simulink model "v2022_Modello_SITL_AENEA_2020b"  (R2020b)
settings: Solver=ode4  StartTime=0.0  StopTime=300  FixedStep=0.01  RelTol=1e-3
values from neighbouring files (symbols this model uses):
  alphavec_rad = [-0.10471975512 -0.0872664625997 -0.0698131700798 -0.0523598775598 -0.0349065850399 -0.0174532925199 0 0.0174532925199 0.0349065850399 0.0523598775598 0.0698131700798 0.0872664625997 ... (13 elements, 1x13)]    [datiAerodinamiciAENEA.mat]    (also in v2021_10_27_calcoloAerodinamica.m = deg2rad(alphavec))
  attuatore_Amax = 20*(pi/180)    (= 0.349065850399)    [v2021_10_27_avvioSITL.m]    (also in v2021_10_27_calcoloAerodinamica.m)
  attuatore_Emax = 25*(pi/180)    (= 0.436332312999)    [v2021_10_27_avvioSITL.m]    (also in v2021_10_27_calcoloAerodinamica.m)
  attuatore_Rmax = 25*(pi/180)    (= 0.436332312999)    [v2021_10_27_avvioSITL.m]    (also in v2021_10_27_calcoloAerodinamica.m)
  b = 2.62    [datiAerodinamiciAENEA.mat]    (also in derivateROSKAM_new.m; v2021_10_27_calcoloAerodinamica.m)
  beta_phi = 1/10.5600    (= 0.094696969697)    [Load_modello_sensori.m]
  beta_psi = 1/170    (= 0.00588235294118)    [Load_modello_sensori.m]
  beta_theta = 1/10.5000    (= 0.0952380952381)    [Load_modello_sensori.m]
  betavec_rad = [-0.209439510239 -0.13962634016 -0.0698131700798 0 0.0698131700798 0.13962634016 0.209439510239]    [datiAerodinamiciAENEA.mat]    (also in v2021_10_27_calcoloAerodinamica.m = deg2rad(betavec))
  c = 0.32    [datiAerodinamiciAENEA.mat]    (also in derivateROSKAM_new.m; v2021_10_27_calcoloAerodinamica.m)
  cbar = 0.32    [datiAerodinamiciAENEA.mat]    (also in v2021_10_27_calcoloAerodinamica.m)
  CD0 = 0.2    [datiAerodinamiciAENEA.mat]    (also in v2021_10_27_calcoloAerodinamica.m = 0.024)
  CldA = KCldA(1)*180/pi    [Alettoni.m]    (also in datiAerodinamiciAENEA.mat = 0.490103315517)
  CLdE = KCLdE(1)*180/pi    [Equilibratore.m]    (also in datiAerodinamiciAENEA.mat = 0.809101149087)
  CldR = 0.0568697125654    [datiAerodinamiciAENEA.mat]
  Clp = -0.4318    [datiAerodinamiciAENEA.mat]    (also in derivateROSKAM_new.m = clp_w+2*(Zv/b)^2*cy_betav+Clp_tail; v2021_10_27_calcoloAerodinamica.m)
  CLq = 8.13    [datiAerodinamiciAENEA.mat]    (also in v2021_10_27_calcoloAerodinamica.m)
  Clr = 0.1459    [datiAerodinamiciAENEA.mat]    (also in derivateROSKAM_new.m = cl*clr_cl-(2/b^2)*(lv*cos(alpha)+Zv*sin(alpha))*(Zv*cos(alph; v2021_10_27_calcoloAerodinamica.m)
  CmdE = KCmdE(1)*180/pi    [Equilibratore.m]    (also in datiAerodinamiciAENEA.mat = -3.59730623976)
  Cmq = -23.24    [datiAerodinamiciAENEA.mat]    (also in derivateROSKAM_new.m = -K*cL_alphaw*((AR*(2*(Xw/c)^2+0.5*(Xw/c))/(AR+2))+1/8)-2*cL_; v2021_10_27_calcoloAerodinamica.m)
  CndA = KCndA(1)*180/pi    [Alettoni.m]    (also in datiAerodinamiciAENEA.mat = -0.0456969018066)
  CndR = -0.162544523826    [datiAerodinamiciAENEA.mat]
  Cnp = 0.000294    [datiAerodinamiciAENEA.mat]    (also in derivateROSKAM_new.m = -clp_w*tan(alpha)+Clp*tan(alpha)-(2/b)*(lv*cos(alpha)+Zv*sin; v2021_10_27_calcoloAerodinamica.m = 0.007507)
  Cnr = -0.4872    [datiAerodinamiciAENEA.mat]    (also in derivateROSKAM_new.m = (Cnr_Clquadro)*cl^2+(cnr_cd0)*cd0+(2/b^2)*(lv*cos(alpha)+Zv*; v2021_10_27_calcoloAerodinamica.m)
  CYdA = KCYdA(1)*180/pi    [Alettoni.m]    (also in datiAerodinamiciAENEA.mat = -0.0146577407549)
  CYdR = -0.298131751664    [datiAerodinamiciAENEA.mat]
  CYp = 0.050728    [datiAerodinamiciAENEA.mat]    (also in v2021_10_27_calcoloAerodinamica.m)
  CYr = 0.358925    [datiAerodinamiciAENEA.mat]    (also in v2021_10_27_calcoloAerodinamica.m)
  delay_ahrs = 0    [Load_modello_sensori.m]
  delay_bmp = 0    [Load_modello_sensori.m]
  delay_gps = 0    [Load_modello_sensori.m]
  deltaAtrim = 0    [v2021_10_27_avvioSITL.m]
  deltaEtrim = (Cm0*CL_alpharad+Cm_alpharad*CLtrim)/(CL_alpharad*CmdE)    [calcoloDatiIniziali.m]    (also in v2021_10_27_avvioSITL.m = 0)
  deltaRtrim = 0    [v2021_10_27_avvioSITL.m]
  deltaTtrim = 0.1    [v2021_10_27_avvioSITL.m]
  Dprop = 0.5334    [datiAerodinamiciAENEA.mat]    (also in v2021_10_27_calcoloAerodinamica.m)
  g = [0 0 9.81]    [datiAerodinamiciAENEA.mat]    (also in v2021_10_27_calcoloAerodinamica.m = [0 0 9.81]')
  HINI = -State0.Pos0(3)    [v2021_10_27_avvioSITL.m]
  Ingaggio_AP = input("inserire 1 se si vuole ingaggiare l' AP, 0 altrimenti: ")    [v2021_10_27_avvioSITL.m]
  J_vec = [0 0.03 0.06 0.09 0.11 0.14 0.17 0.2 0.23 0.26 0.28 0.31 ... (30 elements, 30x1)]    [datiAerodinamiciAENEA.mat]
  Jeng = 0    [datiAerodinamiciAENEA.mat]    (also in v2021_10_27_calcoloAerodinamica.m)
  Jprop = 0.00422031414    [datiAerodinamiciAENEA.mat]    (also in v2021_10_27_calcoloAerodinamica.m)
  latitudineINI = 41.88754294247101*pi/180    (= 0.731075539917)    [v2021_10_27_avvioSITL.m]
  longitudineINI = 12.539364533818434*pi/180    (= 0.218853197223)    [v2021_10_27_avvioSITL.m]
  mean_ax = 0*0.0392    (= 0)    [Load_modello_sensori.m]
  mean_ay = -0*0.0598    (= 0)    [Load_modello_sensori.m]
  mean_az = 0*0.0384    (= 0)    [Load_modello_sensori.m]
  mean_p = 0*1.5184e-06    (= 0)    [Load_modello_sensori.m]
  mean_q = 0*2.9671e-05    (= 0)    [Load_modello_sensori.m]
  mean_r = 0*5.4105e-05    (= 0)    [Load_modello_sensori.m]
  P_ref = 1.0074e+05    (= 100740)    [Load_modello_sensori.m]
  PWM_Aileron = rad2deg(deltaAtrim)*9+1503    [v2021_10_27_avvioSITL.m]
  PWM_Elevator = rad2deg(deltaEtrim)*(447/50)+(3007/2)    [v2021_10_27_avvioSITL.m]
  PWM_Rudder = rad2deg(deltaRtrim)*(447/50)+(3007/2)    [v2021_10_27_avvioSITL.m]
  PWM_Throttle = (deltaTtrim)*800+1100    (= 1180)    [v2021_10_27_avvioSITL.m]
  q = prediction(11)    [f_pred_F1B.m]
  r = prediction(12)    [f_pred_F1B.m]
  rACtG = [-1.334 0 -0.2103]    [datiAerodinamiciAENEA.mat]    (also in v2021_10_27_calcoloAerodinamica.m = rACtP-rGP)
  rACwG = [-0.0589 0 -0.1645]    [datiAerodinamiciAENEA.mat]    (also in v2021_10_27_calcoloAerodinamica.m = rACwP-rGP)
  rAHRSG = [0 0 0.1075]    [datiAerodinamiciAENEA.mat]    (also in v2021_10_27_calcoloAerodinamica.m = rAHRSP-rGP)
  rho = 1.2133    [datiAerodinamiciAENEA.mat]    (also in derivateROSKAM_new.m = 1.16123787958; v2021_10_27_calcoloAerodinamica.m)
  rLEG = [0.0211 0 -0.1645]    [datiAerodinamiciAENEA.mat]    (also in v2021_10_27_calcoloAerodinamica.m = rLEP-rGP)
  rmglG = [-0.2319 -0.2 0.3925]    [datiAerodinamiciAENEA.mat]    (also in v2021_10_27_calcoloAerodinamica.m = rmglP-rGP)
  rmgrG = [-0.2319 0.2 0.3925]    [datiAerodinamiciAENEA.mat]    (also in v2021_10_27_calcoloAerodinamica.m = rmgrP-rGP)
  rngG = [0.2969 0 0.3925]    [datiAerodinamiciAENEA.mat]    (also in v2021_10_27_calcoloAerodinamica.m = rngP-rGP)
  rNPG = [-0.2442 0 -0.1645]    [datiAerodinamiciAENEA.mat]    (also in v2021_10_27_calcoloAerodinamica.m = rNPP-rGP)
  rPG = [0.5 0 -0.1075]    [datiAerodinamiciAENEA.mat]    (also in v2021_10_27_calcoloAerodinamica.m = -rGP)
  Rprop = 0.2667    [datiAerodinamiciAENEA.mat]    (also in v2021_10_27_calcoloAerodinamica.m)
  S = 0.8384    [datiAerodinamiciAENEA.mat]    (also in derivateROSKAM_new.m; v2021_10_27_calcoloAerodinamica.m)
  seed_ahrs = randi([0 2000],1,1)    [Load_modello_sensori.m]
  seed_baro = randi([0 2000],1,1)    [Load_modello_sensori.m]
  seed_gps = randi([0 2000],1,1)    [Load_modello_sensori.m]
  sensori_FreqCampionamento_pitot = 0.02    [v2021_10_27_avvioSITL.m]
  sensori_RumoreSampleTime = 0.02    [v2021_10_27_avvioSITL.m]
  sensori_varianza = 0.0000    (= 0)    [v2021_10_27_avvioSITL.m]
  Std_con_lat = 2.7349e-07    [Load_modello_sensori.m]
  Std_con_long = 1.3733e-06    [Load_modello_sensori.m]
  Std_vel = 0.05    [Load_modello_sensori.m]
  T0_ref = 25    [Load_modello_sensori.m]
  Ta_lat = 10^2    (= 100)    [Load_modello_sensori.m]
  Ta_long = 10^2    (= 100)    [Load_modello_sensori.m]
  Ts_ahrs = 0.02    [Load_modello_sensori.m]
  Ts_bmp = 0.02    [Load_modello_sensori.m]
  Ts_gps = 0.2    [Load_modello_sensori.m]
  tsamp = 0.02    [v2021_10_27_avvioSITL.m]
  V_cruise = input('inserire un valore desiderato per V_cruise: ')    [trimCalc.m]
  Var_heading_static = 0.1    [Load_modello_sensori.m]
  Var_V_hor = 0.5*0.01    (= 0.005)    [Load_modello_sensori.m]
  Var_V_hor_static = 0.25    [Load_modello_sensori.m]
  W = [0 0 92.214]    [datiAerodinamiciAENEA.mat]    (also in derivateROSKAM_new.m = 112.815; v2021_10_27_calcoloAerodinamica.m = m*g)
  White_ax = 1.486e-04    (= 0.0001486)    [Load_modello_sensori.m]
  White_ay = 9.403e-05    [Load_modello_sensori.m]
  White_az = 1.648e-04    (= 0.0001648)    [Load_modello_sensori.m]
  White_gm_phi = 3.2740e-05    (= 3.274e-05)    [Load_modello_sensori.m]
  White_gm_psi = 2.9162e-04    (= 0.00029162)    [Load_modello_sensori.m]
  White_gm_theta = 2.4704e-05    [Load_modello_sensori.m]
  White_p = 2.934e-05    [Load_modello_sensori.m]
  White_pressione = 10.18    [Load_modello_sensori.m]
  White_r = 3.258e-05    [Load_modello_sensori.m]
  WP_AL = [     0 20 0 0 41.807822 12.589274 3 ... (first row only)    [v2021_10_27_avvioSITL.m]
  WP_db_info = [0 0 0 0 1 3;              0 0 0 0 2 3;              0 0 0 0 3 3;              0 0 0 0 0 0]    [v2021_10_27_avvioSITL.m]
  WP_db_param = [              0 0 17 0 41.887798530888304, 12.537905412104232 75;              0 0 20 0 41.89052329007801, 12.492437426923948 65;              0 0 24 0 41.93506891472633, 12.504514543566634 80;              0 0 0 0 0 0 0 ... (first row only)    [v2021_10_27_avvioSITL.m]
  Zeng = -0.1075    [datiAerodinamiciAENEA.mat]    (also in v2021_10_27_calcoloAerodinamica.m = rPG(3))
  Zpista = 0    [v2021_10_27_avvioSITL.m]
undefined symbols (not defined in the file or in its folder): Earth, F, h_home, matricepolinomi, MIL, Receive, Send, State0, Var_heading, WGS84
libraries: simulink_extras x27, aerolibfltsims x5, simulink x3, aerolibwind2 x3, aerolibasang x2, shared6dof x1, slpidlib x1, aerolibatmos2 x1, aerolibanimutils x1
(part 1 of 4)
settings Model: PacingRate=0.010000  Creator=Giorgio  LastModifiedBy=User
settings DataIOCC: ReturnWorkspaceOutputs=off
settings DebuggingCC: ParameterPrecisionLossMsg=none  BusObjectLabelMismatch=none  ArithmeticOperatorsInVariantConditions=warning
settings SFSimCC: CustomCodeUndefinedFunction=UseInterfaceOnly

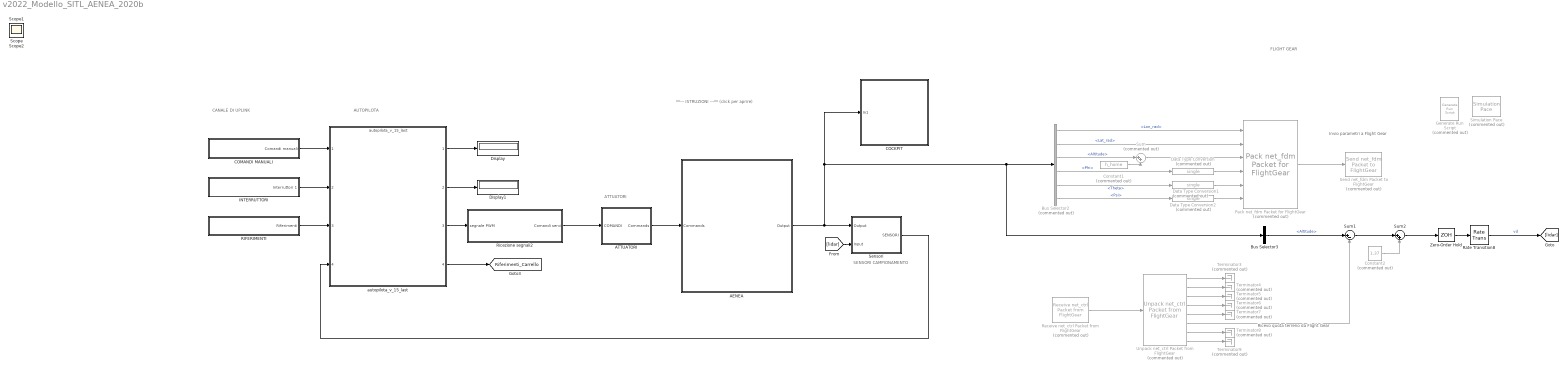
== system v2022_Modello_SITL_AENEA_2020b ==
  note: AUTOPILOTA
  note: SENSORI
      | CAMPIONAMENTO
  note: ATTUATORI
  note: CANALE DI UPLINK
  note: Ricevo quota terreno da Flight Gear
  note: Invio parametri a Flight Gear
  note: FLIGHT GEAR
  note: **--- ISTRUZIONI ---**
      | (click per aprire)
  "AENEA " : Subsystem
  ATTUATORI : Subsystem
  Bus Selector2 : BusSelector  Commented=on  OutputSignals=Lon_rad,Lat_rad,Altitude,Phi,Theta,Psi
  Bus Selector3 : BusSelector  OutputSignals=Altitude
  COCKPIT : Subsystem
  COMANDI MANUALI : Subsystem
  Constant1 : Constant  Commented=on  Value=h_home
  Constant2 : Constant  Commented=on  Value=1.37
  Data Type Conversion : DataTypeConversion  Commented=on  OutDataTypeStr=single
  Data Type Conversion1 : DataTypeConversion  Commented=on  OutDataTypeStr=single
  Data Type Conversion2 : DataTypeConversion  Commented=on  OutDataTypeStr=single
  Display : Display
  Display1 : Display
  Generate Run Script : aerolibfltsims/Generate Run Script  Commented=on  Architecture=Default  dataFlow=Send-Receive  GeometryModelName=c172p  AirportId=LIRF  RunwayId=34L  InitialAltitude=0  InitialHeading=340  OffsetDistance=0  OffsetAzimuth=0  InstallScenery=off  DisableShaders=off  OriginAddress=127.0.0.1  DestinationPort=5502  OriginPort=5505  LocalAddress=127.0.0.1  OutputFileName=runfg_sr.bat  FlightGearBaseDirectory=C:\Program Files\FlightGear 2016.1.2
  "INTERRUTTORI " : Subsystem
  Pack net_fdm Packet for FlightGear : aerolibfltsims/Pack net_fdm Packet for FlightGear  Commented=on  FlightGearVersion=v2016.1  ShowPositionAttitudeInputs=on  ShowVelocityAccelerationInputs=off  ShowControlSurfacePositionInputs=off  ShowEngineFuelInputs=off  ShowLandingGearInputs=off  ShowEnvironmentInputs=off  SampleTime=-1  packetVersion=24
      settings: SourceProductBaseCode=AE
  RIFERIMENTI : Subsystem
  Rate Transition8 : RateTransition  Deterministic=off  InitialCondition=State0.Pos0(3)  OutPortSampleTime=0.02
  Receive net_ctrl Packet from FlightGear : aerolibfltsims/Receive net_ctrl Packet from FlightGear  Commented=on  FlightGearVersion=v2016.1  ReceiveAddress=127.0.0.1  ReceivePort=5505  ReceiveWidth=744  varLen=off  SampleTime=-1  packetFlag=off
      settings: AttributesFormatString=Version Selected:\n%<FlightGearVersion>  SourceProductBaseCode=AE
  Ricezione segnali2 : Subsystem
  Send net_fdm Packet to FlightGear : aerolibfltsims/Send net_fdm Packet to FlightGear  Commented=on  DestinationIpAddress=127.0.0.1  DestinationPort=5502  LocalIpPort=-1  varLen=off  SampleTime=-1
      settings: SourceProductBaseCode=AE
  Sensori : Subsystem
  Simulation Pace : aerolibanimutils/Simulation Pace  Commented=on  SimulationPace=1  SleepMode=MATLAB Thread  OutputPaceError=off  SampleTime=tsamp
  Sum : Sum  Commented=on  Inputs=|++
  Sum1 : Sum  Inputs=|+-
  Sum2 : Sum  Inputs=|++
  Terminator{3..9} (7 alike) : Terminator  Commented=on
  Unpack net_ctrl Packet from FlightGear : aerolibfltsims/Unpack net_ctrl Packet from FlightGear  Commented=on  FlightGearVersion=v2016.1  ShowControlSurfacePositionOutputs=off  ShowEngineFuelOutputs=off  ShowLandingGearOutputs=off  ShowAvionicOutputs=off  ShowEnvironmentOutputs=on  SampleTime=-1  packetVersion=27
      settings: AttributesFormatString=Version Selected: %<FlightGearVersion>  SourceProductBaseCode=AE
  Zero-Order Hold : ZeroOrderHold  SampleTime=0.02
  autopilota_v_15_last : ModelReference  ModelNameDialog=autopilota_v_15_last.slx  SimulationMode=Normal  ModelReferenceVersion=4.21
  Scope : Scope
  Scope1 : Scope
  Scope2 : Scope
  tag scope: Riferimenti_Carrello=global
  wires:
  autopilota_v_15_last/1 -> Display/1
  "INTERRUTTORI "/1(Interruttori 1) -> autopilota_v_15_last/2
  COMANDI MANUALI/1(Comandi manuali) -> autopilota_v_15_last/1
  autopilota_v_15_last/2 -> Display1/1
  RIFERIMENTI/1(Riferimenti) -> autopilota_v_15_last/3
  Constant2/1 -> Sum2/2
  Bus Selector2/6 -> Data Type Conversion2/1  "<Psi>"
  Bus Selector2/3 -> Sum/1  "<Altitude>"
  Sum1/1 -> Sum2/1
  Unpack net_ctrl Packet from FlightGear/6 -> Sum1/2
  Unpack net_ctrl Packet from FlightGear/2 -> Terminator4/1
  Unpack net_ctrl Packet from FlightGear/7 -> Terminator8/1
  Rate Transition8/1 -> [lidar]  "vd"
  Receive net_ctrl Packet from FlightGear/1 -> Unpack net_ctrl Packet from FlightGear/1
  Sum2/1 -> Zero-Order Hold/1
  Unpack net_ctrl Packet from FlightGear/8 -> Terminator9/1
  Bus Selector2/2 -> Pack net_fdm Packet for FlightGear/2  "<Lat_rad>"
  Constant1/1 -> Sum/2
  Data Type Conversion2/1 -> Pack net_fdm Packet for FlightGear/6
  Bus Selector3/1 -> Sum1/1  "<Altitude>"
  Unpack net_ctrl Packet from FlightGear/3 -> Terminator5/1
  Pack net_fdm Packet for FlightGear/1 -> Send net_fdm Packet to FlightGear/1
  Zero-Order Hold/1 -> Rate Transition8/1
  Data Type Conversion/1 -> Pack net_fdm Packet for FlightGear/4
  Sum/1 -> Pack net_fdm Packet for FlightGear/3
  Bus Selector2/4 -> Data Type Conversion/1  "<Phi>"
  Bus Selector2/5 -> Data Type Conversion1/1  "<Theta>"
  Unpack net_ctrl Packet from FlightGear/1 -> Terminator3/1
  Data Type Conversion1/1 -> Pack net_fdm Packet for FlightGear/5
  Bus Selector2/1 -> Pack net_fdm Packet for FlightGear/1  "<Lon_rad>"
  Unpack net_ctrl Packet from FlightGear/4 -> Terminator6/1
  Unpack net_ctrl Packet from FlightGear/5 -> Terminator7/1
  [lidar] -> Sensori/2(Input)
  "AENEA "/1(Output) -> Sensori/1(Output), COCKPIT/1(In1), Bus Selector3/1, Bus Selector2/1
  ATTUATORI/1(Commands) -> "AENEA "/1(Commands)
  autopilota_v_15_last/3 -> Ricezione segnali2/1(segnale PWM)
  Ricezione segnali2/1(Comandi servi) -> ATTUATORI/1("COMANDI ")
  Sensori/1(SENSORI) -> autopilota_v_15_last/4
  autopilota_v_15_last/4 -> [Riferimenti_Carrello]

== system v2022_Modello_SITL_AENEA_2020b/AENEA  ==
  Commands : Inport  OutDataTypeStr=double
  AENEA II_SITL1 : Subsystem
  Blocco_Costanti1 : Subsystem
  Bus Creator : BusCreator  Inputs=4
  Bus Creator1 : BusCreator  Inputs=4
  Bus Selector : BusSelector  OutputSignals=deltaE,deltaA,deltaR,Manetta
  Bus Selector1 : BusSelector  OutputSignals=xyz.h
  Bus Selector2 : BusSelector  OutputSignals=Vbpolare.V
  Constant : Constant  Value=[0,0,0]
  Constant1 : Constant  Value=rho
  Constant2 : Constant  Value=1/2
  Gain : Gain  Gain=-1
  ISA Atmosphere Model : aerolibatmos2/ISA Atmosphere Model  custom=off  g=9.80665  gamma=1.4  R=287.0531  L=0.0065  h_trop=11000  h_strat=20000  rho0=1.225  P0=101325  T0=288.15  h0=0
  Product : Product  Inputs=3
  Square : Math  Operator=square  SaturateOnIntegerOverflow=on
  Terminator : Terminator
  Terminator1 : Terminator
  Terminator2 : Terminator
  toSensors : Subsystem
  Output : Outport  VectorParamsAs1DForOutWhenUnconnected=off
  wires:
  Bus Selector/2 -> Bus Creator/2  "<deltaA>"
  Blocco_Costanti1/1(Vect_Costanti) -> AENEA II_SITL1/2(Vect_Costanti), Bus Creator1/4  "Costanti"
  Bus Creator/1 -> AENEA II_SITL1/1(Vect_Comandi)
  Gain/1 -> ISA Atmosphere Model/1
  Bus Selector/4 -> Bus Creator/4  "<Manetta>"
  Bus Selector/1 -> Bus Creator/1  "<deltaE>"
  Bus Selector/3 -> Bus Creator/3  "<deltaR>"
  ISA Atmosphere Model/2 -> Terminator1/1
  ISA Atmosphere Model/1 -> Terminator2/1
  Constant/1 -> AENEA II_SITL1/4(Constant Wind)  "Constant Wind"
  Commands/1 -> Bus Selector/1
  Bus Selector1/1 -> Gain/1  "<h>"
  Bus Creator1/1 -> toSensors/1("[X,Y,Xpunto,Costanti]")
  AENEA II_SITL1/3(Xpunto) -> Bus Creator1/3  "Xpunto"
  AENEA II_SITL1/1(Xstato) -> Bus Selector1/1, Bus Creator1/1  "X"
  ISA Atmosphere Model/3 -> Terminator/1
  toSensors/1(Out_to_campionamento) -> Output/1
  Constant1/1 -> AENEA II_SITL1/3(ρ)
  Square/1 -> Product/3
  AENEA II_SITL1/2(Y) -> Bus Creator1/2, Bus Selector2/1  "Y"
  Constant2/1 -> Product/2
  Product/1 -> toSensors/3(deltaP)  "deltaP"
  ISA Atmosphere Model/4 -> Product/1, toSensors/2(rho)
  Bus Selector2/1 -> Square/1  "<V>"

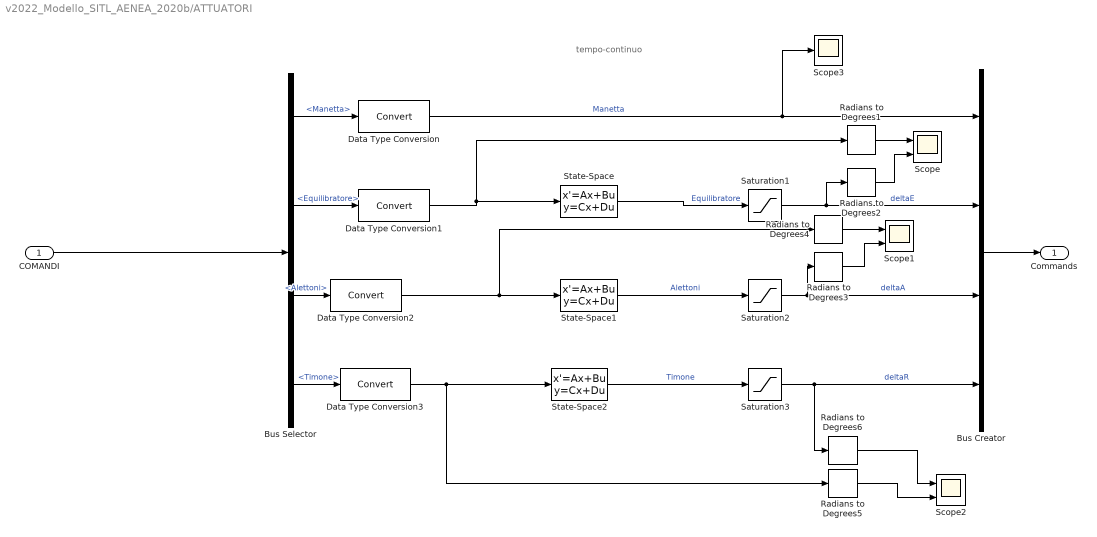
== system v2022_Modello_SITL_AENEA_2020b/ATTUATORI ==
  note: tempo-continuo
  "COMANDI " : Inport
  Bus Creator : BusCreator  Inputs=4
  Bus Selector : BusSelector  OutputSignals=Manetta,Equilibratore,Alettoni,Timone
  Data Type Conversion{,1..3} (4 alike) : DataTypeConversion
  Radians to Degrees{1..6} (6 alike) : simulink_extras/Transformations/Radians to Degrees
  Saturation1 : Saturate  UpperLimit=attuatore_Emax+0.1  LowerLimit=-attuatore_Emax
  Saturation2 : Saturate  UpperLimit=attuatore_Amax+0.1  LowerLimit=-attuatore_Amax
  Saturation3 : Saturate  UpperLimit=attuatore_Rmax+0.1  LowerLimit=-attuatore_Rmax
  Scope : Scope  NumInputPorts=2
  Scope1 : Scope  NumInputPorts=2
  Scope2 : Scope  NumInputPorts=2
  Scope3 : Scope
  State-Space : StateSpace  A=-12.54  C=12.54  D=0  InitialCondition=State0.Ele0
  State-Space1 : StateSpace  A=-12.54  C=12.54  D=0  InitialCondition=State0.Ail0
  State-Space2 : StateSpace  A=-12.54  C=12.54  D=0  InitialCondition=State0.Rud0
  Commands : Outport  VectorParamsAs1DForOutWhenUnconnected=off
  wires:
  "COMANDI "/1 -> Bus Selector/1
  Radians to Degrees3/1 -> Scope1/2
  Bus Selector/2 -> Data Type Conversion1/1  "<Equilibratore>"
  State-Space/1 -> Saturation1/1  "Equilibratore"
  Radians to Degrees1/1 -> Scope/1
  Radians to Degrees4/1 -> Scope1/1
  Saturation2/1 -> Radians to Degrees3/1, Bus Creator/3  "deltaA"
  Saturation1/1 -> Bus Creator/2, Radians to Degrees2/1  "deltaE"
  Bus Selector/1 -> Data Type Conversion/1  "<Manetta>"
  Saturation3/1 -> Radians to Degrees6/1, Bus Creator/4  "deltaR"
  Bus Creator/1 -> Commands/1
  Radians to Degrees6/1 -> Scope2/1
  Bus Selector/3 -> Data Type Conversion2/1  "<Alettoni>"
  Radians to Degrees2/1 -> Scope/2
  Bus Selector/4 -> Data Type Conversion3/1  "<Timone>"
  State-Space2/1 -> Saturation3/1  "Timone"
  State-Space1/1 -> Saturation2/1  "Alettoni"
  Radians to Degrees5/1 -> Scope2/2
  Data Type Conversion/1 -> Scope3/1, Bus Creator/1  "Manetta"
  Data Type Conversion1/1 -> State-Space/1, Radians to Degrees1/1
  Data Type Conversion2/1 -> State-Space1/1, Radians to Degrees4/1
  Data Type Conversion3/1 -> State-Space2/1, Radians to Degrees5/1

== system v2022_Modello_SITL_AENEA_2020b/COCKPIT ==
  In1 : Inport
  Bus Selector : BusSelector  OutputSignals=α,β,V,Lat_rad,Lon_rad,Altitude,Phi,Theta,Psi,p,q,r,upunto,vpunto,wpunto,heading,Xepunto,Yepunto,Zepunto
  Radians to Degrees : simulink_extras/Transformations/Radians to Degrees
  Radians to Degrees1 : simulink_extras/Transformations/Radians to Degrees
  Terminator{,1..18} (19 alike) : Terminator
  wires:
  In1/1 -> Bus Selector/1
  Bus Selector/1 -> Terminator/1  "<α>"
  Bus Selector/2 -> Terminator1/1  "<β>"
  Bus Selector/3 -> Terminator2/1  "<V>"
  Bus Selector/4 -> Radians to Degrees/1  "<Lat_rad>"
  Bus Selector/5 -> Radians to Degrees1/1  "<Lon_rad>"
  Bus Selector/6 -> Terminator5/1  "<Altitude>"
  Bus Selector/7 -> Terminator6/1  "<Phi>"
  Bus Selector/8 -> Terminator7/1  "<Theta>"
  Bus Selector/9 -> Terminator8/1  "<Psi>"
  Bus Selector/10 -> Terminator9/1  "<p>"
  Bus Selector/11 -> Terminator10/1  "<q>"
  Bus Selector/12 -> Terminator11/1  "<r>"
  Bus Selector/13 -> Terminator13/1  "<upunto>"
  Bus Selector/14 -> Terminator12/1  "<vpunto>"
  Bus Selector/15 -> Terminator14/1  "<wpunto>"
  Bus Selector/16 -> Terminator15/1  "<heading>"
  Bus Selector/17 -> Terminator16/1  "<Xepunto>"
  Bus Selector/18 -> Terminator17/1  "<Yepunto>"
  Bus Selector/19 -> Terminator18/1  "<Zepunto>"
  Radians to Degrees1/1 -> Terminator4/1  "Lon_deg"
  Radians to Degrees/1 -> Terminator3/1  "Lat_deg"

== system v2022_Modello_SITL_AENEA_2020b/COMANDI MANUALI ==
  A : Constant  Value=deltaAtrim  SampleTime=0.02
  Bus Creator3 : BusCreator  Inputs=5  OutDataTypeStr=Bus: slBus4_manuali
  Chart : Stateflow chart  TreatAsAtomicUnit=on
  Clock8 : Clock
  Constant : Constant
  Constant1 : Constant  Value=0
  Constant2 : Constant
  E : Constant  Value=deltaEtrim  SampleTime=0.02
  Manual Switch : ManualSwitch  CurrentSetting=0
  R : Constant  Value=deltaRtrim  SampleTime=0.02
  Switch : Switch  Criteria=u2 > Threshold  Threshold=1500
  T : Constant  Value=deltaTtrim  SampleTime=0.02
  Comandi manuali : Outport  VectorParamsAs1DForOutWhenUnconnected=off
  wires:
  A/1 -> Bus Creator3/2  "Manual_Aileron"
  E/1 -> Bus Creator3/1  "Manual_Elevator"
  T/1 -> Bus Creator3/4  "Manual_Throttle"
  Constant/1 -> Switch/1
  Constant1/1 -> Switch/3
  Switch/1 -> Bus Creator3/5  "Go_Home"
  Bus Creator3/1 -> Comandi manuali/1  "Comandi manuali"
  R/1 -> Bus Creator3/3  "Manual_Rudder"
  Chart/1(data1) -> Manual Switch/1
  Clock8/1 -> Chart/1(data)
  Manual Switch/1 -> Switch/2
  Constant2/1 -> Manual Switch/2

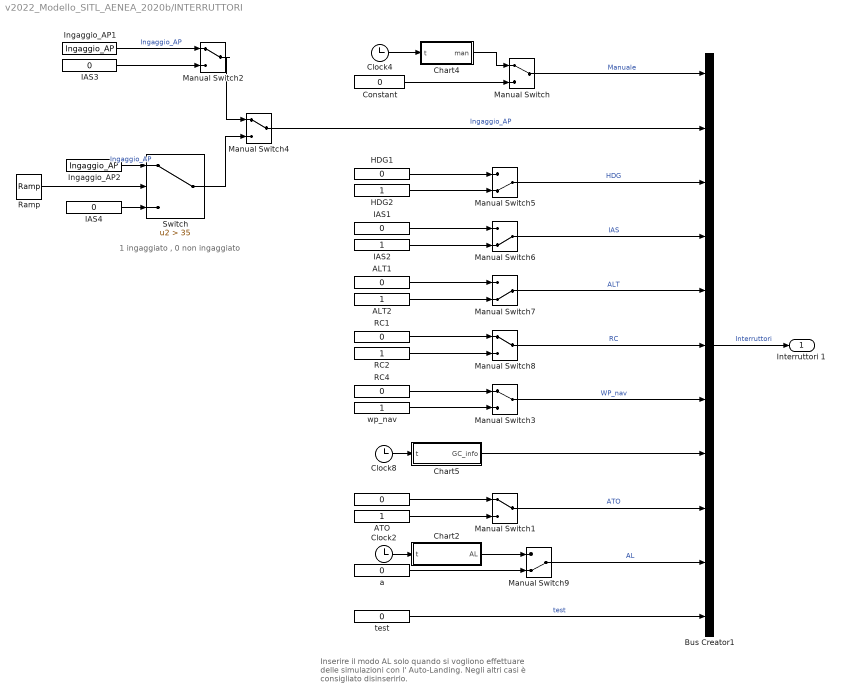
== system v2022_Modello_SITL_AENEA_2020b/INTERRUTTORI  ==
  note: 1 ingaggiato , 0 non ingaggiato
  note: Inserire il modo AL solo quando si vogliono effettuare
      | delle simulazioni con l' Auto-Landing. Negli altri casi è
      | consigliato disinserirlo.
  " " : Constant  Value=0
  ALT1 : Constant  Value=0
  ALT2 : Constant
  ATO : Constant
  Bus Creator1 : BusCreator  Inputs=11
  Chart2 : Stateflow chart  TreatAsAtomicUnit=on
  "Chart4 " : Stateflow chart  TreatAsAtomicUnit=on
  Chart5 : Stateflow chart  TreatAsAtomicUnit=on
  Clock2 : Clock
  Clock4 : Clock
  Clock8 : Clock
  Constant : Constant  Value=0
  HDG1 : Constant  Value=0
  HDG2 : Constant
  IAS1 : Constant  Value=0
  IAS2 : Constant
  IAS3 : Constant  Value=0
  IAS4 : Constant  Value=0
  Ingaggio_AP1 : Constant  Value=Ingaggio_AP
  Ingaggio_AP2 : Constant  Value=Ingaggio_AP
  Manual Switch{,1..4,8} (6 alike) : ManualSwitch
  Manual Switch{5..7,9} (4 alike) : ManualSwitch  CurrentSetting=0
  RC1 : Constant  Value=0
  RC2 : Constant
  RC4 : Constant  Value=0
  Ramp : simulink/Sources/Ramp  slope=1  start=0  InitialOutput=0
  Switch : Switch  Criteria=u2 > Threshold  Threshold=35
  a : Constant  Value=0
  test : Constant  Value=0
  wp_nav : Constant
  Interruttori 1 : Outport  VectorParamsAs1DForOutWhenUnconnected=off
  wires:
  Manual Switch4/1 -> Bus Creator1/2  "Ingaggio_AP"
  Bus Creator1/1 -> Interruttori 1/1  "Interruttori"
  Manual Switch7/1 -> Bus Creator1/5  "ALT"
  Manual Switch6/1 -> Bus Creator1/4  "IAS"
  Manual Switch5/1 -> Bus Creator1/3  "HDG"
  Clock8/1 -> Chart5/1(t)
  Chart5/1(GC_info) -> Bus Creator1/8
  Manual Switch3/1 -> Bus Creator1/7  "WP_nav"
  Manual Switch8/1 -> Bus Creator1/6  "RC"
  test/1 -> Bus Creator1/11  "test"
  Manual Switch1/1 -> Bus Creator1/9  "ATO"
  IAS1/1 -> Manual Switch6/1
  IAS2/1 -> Manual Switch6/2
  HDG2/1 -> Manual Switch5/2
  HDG1/1 -> Manual Switch5/1
  RC4/1 -> Manual Switch3/1
  wp_nav/1 -> Manual Switch3/2
  RC2/1 -> Manual Switch8/2
  RC1/1 -> Manual Switch8/1
  ALT1/1 -> Manual Switch7/1
  Manual Switch9/1 -> Bus Creator1/10  "AL"
  ALT2/1 -> Manual Switch7/2
  Clock4/1 -> "Chart4 "/1(t)
  Manual Switch/1 -> Bus Creator1/1  "Manuale"
  "Chart4 "/1(man) -> Manual Switch/1
  ATO/1 -> Manual Switch1/2
  " "/1 -> Manual Switch1/1
  a/1 -> Manual Switch9/2
  Clock2/1 -> Chart2/1(t)
  Chart2/1(AL) -> Manual Switch9/1
  Constant/1 -> Manual Switch/2
  Ingaggio_AP1/1 -> Manual Switch2/1  "Ingaggio_AP"
  IAS3/1 -> Manual Switch2/2
  Manual Switch2/1 -> Manual Switch4/1
  Switch/1 -> Manual Switch4/2
  Ingaggio_AP2/1 -> Switch/1  "Ingaggio_AP"
  IAS4/1 -> Switch/3
  Ramp/1 -> Switch/2

== system v2022_Modello_SITL_AENEA_2020b/RIFERIMENTI ==
  Bus Creator1 : BusCreator  Inputs=7
  Chart : Stateflow chart  TreatAsAtomicUnit=on
  Chart1 : Stateflow chart  TreatAsAtomicUnit=on
  Chart2 : Stateflow chart  TreatAsAtomicUnit=on
  Clock1 : Clock
  Clock2 : Clock
  Clock3 : Clock
  Manual Switch : ManualSwitch  CurrentSetting=0
  Manual Switch1 : ManualSwitch
  Manual Switch2 : ManualSwitch  CurrentSetting=0
  QUOTA (m) : Constant  Value=80
  RC (ft/min) : Constant  Value=0
  ROTTA  ( ° ) : Constant  Value=0
  VELOCITA'  (m/s) : Constant  Value=25
  WP_AL : Constant  Value=WP_AL
  WP_db_info : Constant  Value=WP_db_info
  WP_db_param : Constant  Value=WP_db_param
  ft/min2m/s : Gain  Gain=0.00508
  Riferimenti : Outport  VectorParamsAs1DForOutWhenUnconnected=off
  wires:
  VELOCITA'  (m/s)/1 -> Manual Switch2/2  "VELOCITA"
  Bus Creator1/1 -> Riferimenti/1  "Riferimenti"
  RC (ft/min)/1 -> ft/min2m/s/1  "RC"
  WP_db_info/1 -> Bus Creator1/5  "WP_db_info"
  WP_db_param/1 -> Bus Creator1/6  "WP_db_param"
  Clock2/1 -> Chart2/1(t)
  Chart2/1(ROTTA) -> Manual Switch/1  "ROTTA"
  Clock1/1 -> Chart1/1(t)
  Chart1/1(QUOTA) -> Manual Switch1/1
  ROTTA  ( ° )/1 -> Manual Switch/2  "ROTTA"
  Manual Switch/1 -> Bus Creator1/1  "ROTTA"
  QUOTA (m)/1 -> Manual Switch1/2  "QUOTA"
  Manual Switch1/1 -> Bus Creator1/3  "QUOTA"
  WP_AL/1 -> Bus Creator1/7  "WP_AL"
  Manual Switch2/1 -> Bus Creator1/2  "VELOCITA"
  ft/min2m/s/1 -> Bus Creator1/4
  Clock3/1 -> Chart/1(t)
  Chart/1(vel) -> Manual Switch2/1

== system v2022_Modello_SITL_AENEA_2020b/Ricezione segnali2 ==
  segnale PWM : Inport
  Bus Creator3 : BusCreator  Inputs=4
  Delay : Delay  InitialCondition=PWM_Throttle
  Delay1 : Delay  InitialCondition=PWM_Elevator
  Delay2 : Delay  InitialCondition=PWM_Aileron
  Delay3 : Delay  InitialCondition=PWM_Rudder
  Demux : Demux
  Display : Display
  Subsystem1 : Subsystem  TreatAsAtomicUnit=on  SystemSampleTime=0.01
  Comandi servi : Outport  VectorParamsAs1DForOutWhenUnconnected=off
  wires:
  segnale PWM/1 -> Demux/1
  Bus Creator3/1 -> Comandi servi/1  "Comandi manuali"
  Demux/1 -> Delay/1
  Demux/2 -> Delay1/1
  Demux/3 -> Delay2/1
  Demux/4 -> Delay3/1
  Subsystem1/1(Out1) -> Bus Creator3/1
  Subsystem1/3(Out3) -> Bus Creator3/3
  Subsystem1/4(Out4) -> Bus Creator3/4
  Delay/1 -> Subsystem1/1(In1)
  Delay1/1 -> Subsystem1/2(In2)
  Delay2/1 -> Subsystem1/3(In3)
  Delay3/1 -> Subsystem1/4(In4)
  Subsystem1/2(Out2) -> Display/1, Bus Creator3/2

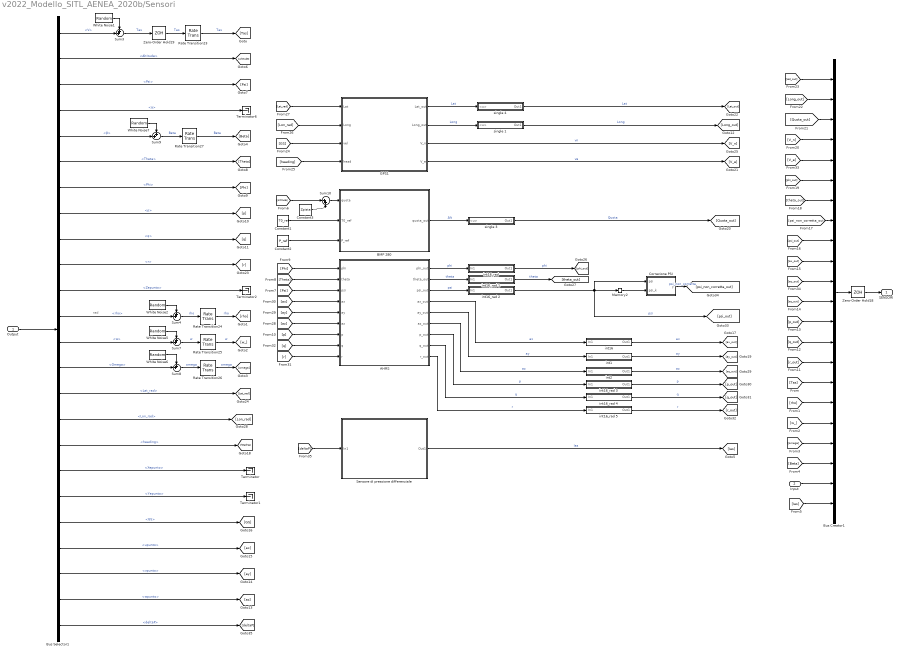
== system v2022_Modello_SITL_AENEA_2020b/Sensori ==
  note: rad
  Output : Inport
  Input : Inport  Port=2
  AHRS : Subsystem
  BMP 280 : Subsystem
  Bus Creator1 : BusCreator  Inputs=22  OutDataTypeStr=Bus: slBus8_sensori2
  Bus Selector1 : BusSelector  OutputSignals=V,Altitude,Psi,α,β,Theta,Phi,p,q,r,Zepunto,rho,w,Omega,Lat_rad,Lon_rad,heading,Xepunto,Yepunto,GS,upunto,vpunto,wpunto,deltaP
  Constant1 : Constant  Value=T0_ref
  Constant2 : Constant  Value=P_ref
  Constant3 : Constant  Value=Zpista
  Correzione PSI : MATLAB Function  TreatAsAtomicUnit=on
  GPS1 : Subsystem
  Memory2 : Memory
  Rate Transition23 : RateTransition  OutPortSampleTime=0.02
  Rate Transition{24..27} (4 alike) : RateTransition  OutPortSampleTimeOpt=Inherit
  Sensore di pressione differenziale : Subsystem
  Sum10 : Sum  Inputs=|++
  Sum{3..4,7..9} (5 alike) : Sum  Inputs=++|
  Terminator{,1..2,6} (4 alike) : Terminator
  White Noise1 : RandomNumber  DisableCoverage=on  Variance=1e-1  Seed=[23341]  SampleTime=sensori_RumoreSampleTime
  White Noise{2,5..7} (4 alike) : RandomNumber  DisableCoverage=on  Variance=sensori_varianza  Seed=[23341]  SampleTime=sensori_RumoreSampleTime
  Zero-Order Hold18 : ZeroOrderHold  SampleTime=0.02
  Zero-Order Hold19 : ZeroOrderHold  SampleTime=sensori_FreqCampionamento_pitot
  int1 : Subsystem
  int16 : Subsystem
  "int16_rad " : Subsystem
  int16_rad 1 : Subsystem
  int16_rad 2 : Subsystem
  int16_rad 3 : Subsystem
  int16_rad 4 : Subsystem
  int16_rad 5 : Subsystem
  int2 : Subsystem
  single 1 : Subsystem
  single 3 : Subsystem
  single 4 : Subsystem
  SENSORI : Outport  OutDataTypeStr=double  VectorParamsAs1DForOutWhenUnconnected=off
  wires:
  GPS1/3(V_n) -> [V_n]  "vn"
  Bus Selector1/19 -> Terminator1/1  "<Yepunto>"
  Bus Selector1/6 -> [Theta]  "<Theta>"
  Bus Selector1/4 -> Terminator6/1  "<α>"
  Bus Selector1/18 -> Terminator/1  "<Xepunto>"
  Bus Selector1/2 -> [Altitude]  "<Altitude>"
  Bus Selector1/17 -> [heading]  "<heading>"
  Bus Selector1/7 -> [Phi]  "<Phi>"
  GPS1/1(Lat_out) -> single 4/1(<u>)  "Lat"
  Rate Transition27/1 -> [Beta]  "Beta"
  "int16_rad "/1(Out1) -> [phi_out]  "phi"
  Bus Selector1/5 -> Sum9/2  "<β>"
  White Noise2/1 -> Sum4/1
  White Noise5/1 -> Sum7/1
  AHRS/7(p_out) -> int16_rad 3/1(In1)  "p"
  Sum4/1 -> Rate Transition24/1  "rho"
  int16/1(Out1) -> [ax_out]  "ax"
  Bus Selector1/14 -> Sum8/2  "<Omega>"
  BMP 280/1(quota_out) -> single 3/1(<u>)  "Alt"
  AHRS/4(ax_out) -> int16/1(In1)  "ax"
  Rate Transition25/1 -> [w_]  "w"
  int16_rad 5/1(Out1) -> [r_out]  "r"
  AHRS/6(az_out) -> int2/1(In1)  "az"
  GPS1/4(V_e) -> [V_e]  "ve"
  Bus Selector1/12 -> Sum4/2  "<rho>"
  Constant1/1 -> BMP 280/2(T0_ref)
  Bus Selector1/8 -> [p]  "<p>"
  Sum7/1 -> Rate Transition25/1  "w"
  Output/1 -> Bus Selector1/1
  Sum3/1 -> Zero-Order Hold19/1  "Tas"
  Bus Selector1/11 -> Terminator2/1  "<Zepunto>"
  AHRS/1(phi_out) -> "int16_rad "/1(In1)  "phi"
  Bus Selector1/9 -> [q]  "<q>"
  Bus Selector1/3 -> [Psi]  "<Psi>"
  int16_rad 3/1(Out1) -> [p_out]  "p"
  Rate Transition23/1 -> [Tas]  "Tas"
  AHRS/9(r_out) -> int16_rad 5/1(In1)  "r"
  int16_rad 4/1(Out1) -> [q_out]  "q"
  White Noise1/1 -> Sum3/1
  int2/1(Out1) -> [az_out]  "az"
  Bus Selector1/20 -> [GS]  "<GS>"
  Memory2/1 -> Correzione PSI/2(psi_k)
  White Noise6/1 -> Sum8/1
  Zero-Order Hold19/1 -> Rate Transition23/1  "Tas"
  AHRS/2(theta_out) -> int16_rad 1/1(In1)  "theta"
  AHRS/8(q_out) -> int16_rad 4/1(In1)  "q"
  int1/1(Out1) -> [ay_out]  "ay"
  single 3/1(Out1) -> [Quota_out]  "Quota"
  GPS1/2("Long_out ") -> single 1/1(<u>)  "Long"
  AHRS/5(ay_out) -> int1/1(In1)  "ay"
  single 1/1(Out1) -> [Long_out]  "Long"
  Rate Transition24/1 -> [rho]  "rho"
  White Noise7/1 -> Sum9/1
  Sum10/1 -> BMP 280/1(quota)
  Bus Selector1/15 -> [Lat_rad]  "<Lat_rad>"
  Constant2/1 -> BMP 280/3(P_ref)
  Rate Transition26/1 -> [omega]  "omega"
  Bus Selector1/1 -> Sum3/2  "<V>"
  Bus Selector1/13 -> Sum7/2  "<w>"
  Sum8/1 -> Rate Transition26/1  "omega"
  int16_rad 1/1(Out1) -> [theta_out]  "theta"
  Sum9/1 -> Rate Transition27/1  "Beta"
  AHRS/3(psi_out) -> int16_rad 2/1(In1)  "psi"
  Zero-Order Hold18/1 -> SENSORI/1
  int16_rad 2/1(Out1) -> Correzione PSI/1(psi), [psi_out], Memory2/1  "psi"
  Constant3/1 -> Sum10/2
  single 4/1(Out1) -> [Lat_out]  "Lat"
  [w_] -> Bus Creator1/18
  [omega] -> Bus Creator1/19
  [Beta] -> Bus Creator1/20
  Input/1 -> Bus Creator1/21
  Bus Creator1/1 -> Zero-Order Hold18/1
  Correzione PSI/1(y) -> [psi_non_corretta_out]  "psi_non_corretta"
  Sensore di pressione differenziale/1(Out1) -> [Ias]  "Ias"
  Bus Selector1/24 -> [deltaP]  "<deltaP>"
  [Ias] -> Bus Creator1/22
  [Altitude] -> Sum10/1
  [Psi] -> AHRS/3(psi)
  [Theta] -> AHRS/2(theta)
  [Phi] -> AHRS/1(phi)
  [p] -> AHRS/7(p)
  [q] -> AHRS/8(q)
  [r] -> AHRS/9(r)
  [ax] -> AHRS/4(ax)
  [ay] -> AHRS/5(ay)
  [az] -> AHRS/6(az)
  Bus Selector1/10 -> [r]  "<r>"
  [Lat_rad] -> GPS1/1(Lat)
  [Lon_rad] -> GPS1/2(Long)
  Bus Selector1/16 -> [Lon_rad]  "<Lon_rad>"
  [heading] -> GPS1/4(head)
  [GS] -> GPS1/3(vel)
  Bus Selector1/21 -> [ax]  "<upunto>"
  Bus Selector1/22 -> [ay]  "<vpunto>"
  Bus Selector1/23 -> [az]  "<wpunto>"
  [Lat_out] -> Bus Creator1/1
  [Long_out] -> Bus Creator1/2
  [Quota_out] -> Bus Creator1/3
  [V_n] -> Bus Creator1/4
  [V_e] -> Bus Creator1/5
  [phi_out] -> Bus Creator1/6
  [theta_out] -> Bus Creator1/7
  [psi_non_corretta_out] -> Bus Creator1/8
  [psi_out] -> Bus Creator1/9
  [ax_out] -> Bus Creator1/10
  [ay_out] -> Bus Creator1/11
  [az_out] -> Bus Creator1/12
  [p_out] -> Bus Creator1/13
  [q_out] -> Bus Creator1/14
  [r_out] -> Bus Creator1/15
  [Tas] -> Bus Creator1/16
  [rho] -> Bus Creator1/17
  [deltaP] -> Sensore di pressione differenziale/1(In1)

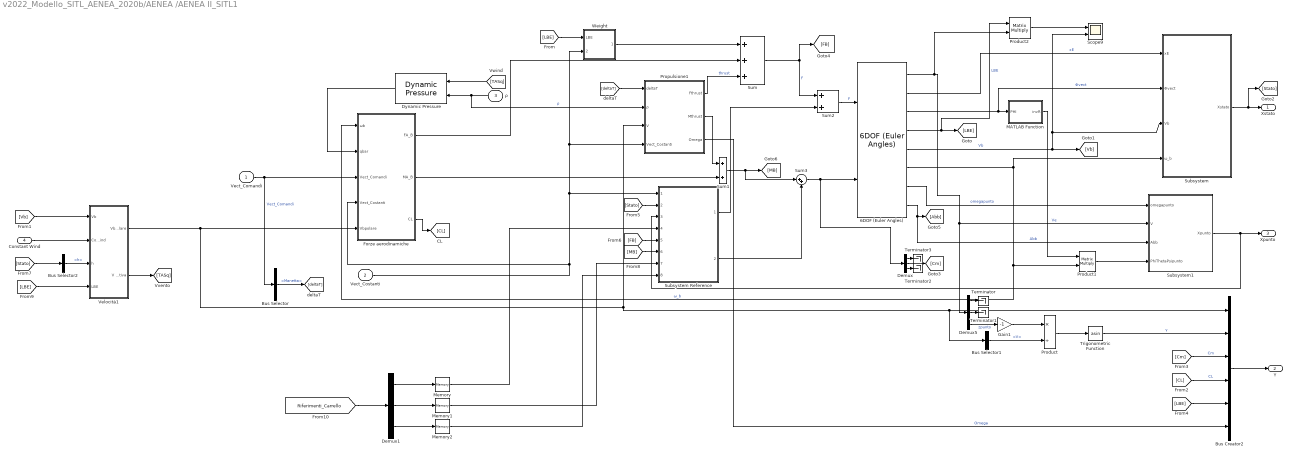
== system v2022_Modello_SITL_AENEA_2020b/AENEA /AENEA II_SITL1 ==
  Vect_Comandi : Inport
  Vect_Costanti : Inport  Port=2
  ρ : Inport  Port=3
  Constant Wind : Inport  Port=4
  6DOF (Euler Angles) : shared6dof/6DOF (Euler Angles)  units=Metric (MKS)  mtype=Fixed  rep=Euler Angles  xme_0=State0.Pos0  Vm_0=State0.Vb0  eul_0=State0.PHI0  pm_0=State0.Omega0  mass_0=m  mass_e=0.5  mass_f=2.0  inertia=I  inertia_e=eye(3)  inertia_f=2*eye(3)  k_quat=1.0  vre_flag=on  abi_flag=off  aMode=aMode  xme_statename=''  Vm_statename=''  eul_statename=''  quat_statename=''  pm_statename=''  mass_statename=''
      settings: SourceProductBaseCode=AE,PW,DR,MT,VE
  Bus Creator2 : BusCreator  Inputs=6
  Bus Selector : BusSelector  OutputSignals=Manetta
  Bus Selector1 : BusSelector  OutputSignals=V
  Bus Selector2 : BusSelector  OutputSignals=xyz.h
  Demux : Demux  Outputs=3
  Demux1 : Demux  Outputs=3
  Demux5 : Demux  Outputs=3
  Dynamic Pressure : aerolibasang/Dynamic Pressure
  Forze aerodinamiche : Subsystem
  Gain1 : Gain  Gain=-1
  MATLAB Function : MATLAB Function  TreatAsAtomicUnit=on
  Memory : Memory
  Memory1 : Memory
  Memory2 : Memory
  Product : Product  Inputs=*/
  Product1 : Product  Multiplication=Matrix(*)
  Product2 : Product  Multiplication=Matrix(*)  InputSameDT=on  RndMeth=Zero  SaturateOnIntegerOverflow=on  OutDataTypeStr=Inherit: Same as first input
  Propulsione1 : Subsystem
  Scope9 : Scope  NumInputPorts=2
  Subsystem : Subsystem
  Subsystem Reference : Subsystem  ReferencedSubsystem=v2021_10_27_Gear
  Subsystem1 : Subsystem
  Sum : Sum  Inputs=+++
  Sum1 : Sum
  Sum2 : Sum
  Sum3 : Sum  Inputs=|++
  Terminator{,1..3} (4 alike) : Terminator
  Trigonometric Function : Trigonometry  Operator=asin
  Velocità1 : Subsystem
  Weight : Subsystem
  Xstato : Outport  VectorParamsAs1DForOutWhenUnconnected=off
  Y : Outport  Port=2  VectorParamsAs1DForOutWhenUnconnected=off
  Xpunto : Outport  Port=3  VectorParamsAs1DForOutWhenUnconnected=off
  wires:
  Sum/1 -> Sum2/1, [FB]  "F"
  6DOF (Euler Angles)/5 -> Scope9/2, Subsystem/3(Vb), [Vb]  "Vb"
  6DOF (Euler Angles)/6 -> Forze aerodinamiche/1(ωb), Product1/2, Subsystem/4(ω_b)  "ω_b"
  6DOF (Euler Angles)/4 -> Product2/1, [LBE]  "LBE"
  Forze aerodinamiche/1(FA_B) -> Sum/2
  Forze aerodinamiche/2(MA_B) -> Sum1/2
  6DOF (Euler Angles)/1 -> Product2/2, Demux5/1, Subsystem1/2(V)  "Ve"
  Dynamic Pressure/1 -> Forze aerodinamiche/2(qbar)
  Sum1/1 -> Sum3/1, [MB]
  Weight/1("Forzapeso ") -> Sum/1
  [LBE] -> Weight/1(LBE)
  Vect_Comandi/1 -> Bus Selector/1, Forze aerodinamiche/3(Vect_Comandi)  "Vect_Comandi"
  Bus Selector/1 -> [deltaT]  "<Manetta>"
  Bus Creator2/1 -> Y/1
  Gain1/1 -> Product/1
  Product/1 -> Trigonometric Function/1
  Trigonometric Function/1 -> Bus Creator2/2  "γ"
  ρ/1 -> Propulsione1/2(ρ), Dynamic Pressure/2  "ρ"
  Velocità1/1(Vbpolare) -> Propulsione1/3(V), Bus Selector1/1, Bus Creator2/1, Forze aerodinamiche/5("Vbpolare ")
  [Vb] -> Velocità1/1(Vb)
  6DOF (Euler Angles)/3 -> Subsystem/2(Φvect), MATLAB Function/1(PHI)  "Φvect"
  Bus Selector1/1 -> Product/2  "<V>"
  Constant Wind/1 -> Velocità1/2(Constant Wind)
  Forze aerodinamiche/3(CL) -> [CL]
  [Cm] -> Bus Creator2/3  "Cm"
  [CL] -> Bus Creator2/4  "CL"
  6DOF (Euler Angles)/2 -> Subsystem/1(xE)  "xE"
  Subsystem/1("Xstato ") -> [Stato], Xstato/1
  Demux5/2 -> Terminator1/1
  Demux5/1 -> Terminator/1
  Demux5/3 -> Gain1/1  "zpunto"
  6DOF (Euler Angles)/7 -> Subsystem1/1(omegapunto)  "omegapunto"
  6DOF (Euler Angles)/8 -> [Abb], Subsystem1/3(Abb)  "Abb"
  Subsystem1/1(Xpunto) -> Xpunto/1, Subsystem Reference/3
  Product1/1 -> Subsystem1/4("PhiThetaPsipunto ")
  MATLAB Function/1(invR) -> Product1/1
  [deltaT] -> Propulsione1/1("deltaT ")
  Vect_Costanti/1 -> Forze aerodinamiche/4(Vect_Costanti), Subsystem Reference/1, Weight/2(Vect_Costanti), Propulsione1/4(Vect_Costanti)
  Propulsione1/2(Mthrust) -> Sum1/1
  Propulsione1/1("Fthrust ") -> Sum/3  "thrust"
  Demux/2 -> [Cm]
  Demux/3 -> Terminator2/1
  Demux/1 -> Terminator3/1
  [LBE] -> Bus Creator2/5
  Propulsione1/3(Omega) -> Bus Creator2/6  "Omega"
  Velocità1/2("V effettiva ") -> [TASq]
  [TASq] -> Dynamic Pressure/1
  Sum2/1 -> 6DOF (Euler Angles)/1  "F"
  [FB] -> Subsystem Reference/5
  Subsystem Reference/1 -> Sum2/2
  Subsystem Reference/2 -> Sum3/2
  Sum3/1 -> Demux/1, 6DOF (Euler Angles)/2
  [MB] -> Subsystem Reference/6
  [Stato] -> Subsystem Reference/2
  [Stato] -> Bus Selector2/1
  Bus Selector2/1 -> Velocità1/3(h)  "<h>"
  [LBE] -> Velocità1/4(LBE)
  Product2/1 -> Scope9/1
  Demux1/3 -> Memory2/1
  Memory2/1 -> Subsystem Reference/8
  [Riferimenti_Carrello] -> Demux1/1
  Demux1/1 -> Memory/1
  Demux1/2 -> Memory1/1
  Memory/1 -> Subsystem Reference/4
  Memory1/1 -> Subsystem Reference/7

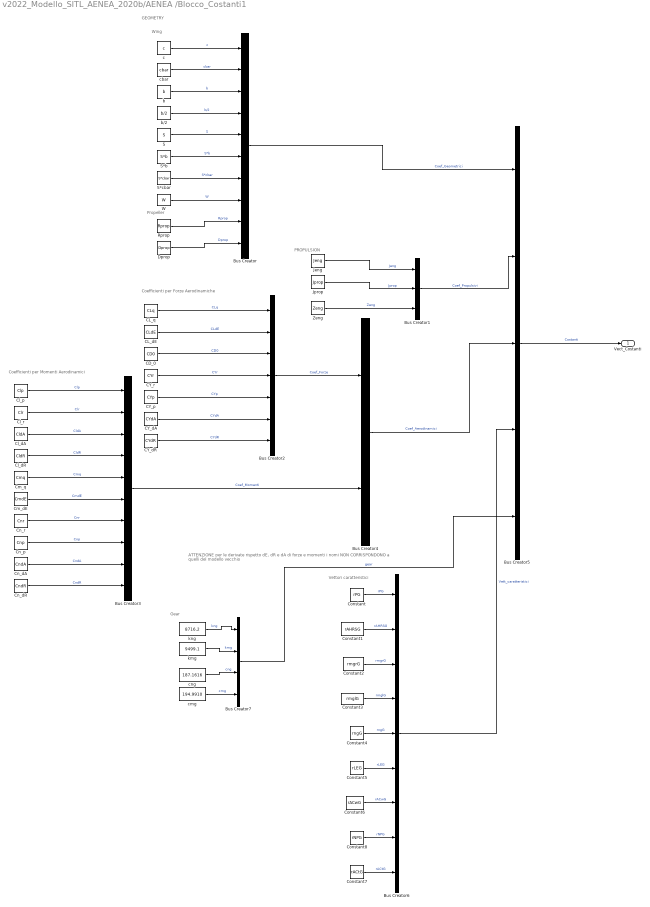
== system v2022_Modello_SITL_AENEA_2020b/AENEA /Blocco_Costanti1 ==
  note: Gear
  note: Vettori caratteristici
  note: ATTENZIONE per le derivate rispetto dE, dR e dA di forze e momenti i nomi NON CORRISPONDONO a quelli del modello vecchio
  note: Coefficienti per Forze Aerodinamiche
  note: Coefficienti per Momenti Aerodinamici
  note: Wing
  note: Propeller
  note: PROPULSION
  note: GEOMETRY
  Bus Creator : BusCreator  Inputs=10
  Bus Creator1 : BusCreator  Inputs=3
  Bus Creator2 : BusCreator  Inputs=7
  Bus Creator3 : BusCreator  Inputs=10
  Bus Creator4 : BusCreator  Inputs=2
  Bus Creator5 : BusCreator  Inputs=5
  Bus Creator6 : BusCreator  Inputs=9
  Bus Creator7 : BusCreator  Inputs=4
  CD_0 : Constant  Value=CD0
  "CL_dE " : Constant  Value=CLdE
  "CL_q " : Constant  Value=CLq
  CY_dA : Constant  Value=CYdA
  CY_dR : Constant  Value=CYdR
  "CY_p " : Constant  Value=CYp
  CY_r : Constant  Value=CYr
  Cl_dA : Constant  Value=CldA
  Cl_dR : Constant  Value=CldR
  "Cl_p " : Constant  Value=Clp
  "Cl_r " : Constant  Value=Clr
  "Cm_dE " : Constant  Value=CmdE
  "Cm_q " : Constant  Value=Cmq
  Cn_dA : Constant  Value=CndA
  "Cn_dR " : Constant  Value=CndR
  "Cn_p " : Constant  Value=Cnp
  "Cn_r " : Constant  Value=Cnr
  Constant : Constant  Value=rPG
  Constant1 : Constant  Value=rAHRSG
  Constant2 : Constant  Value=rmgrG
  Constant3 : Constant  Value=rmglG
  Constant4 : Constant  Value=rngG
  Constant5 : Constant  Value=rLEG
  Constant6 : Constant  Value=rACwG
  Constant7 : Constant  Value=rACtG
  Constant8 : Constant  Value=rNPG
  Dprop : Constant  Value=Dprop
  Jeng : Constant  Value=Jeng
  Jprop : Constant  Value=Jprop
  Rprop : Constant  Value=Rprop
  S : Constant  Value=S
  "S*b " : Constant  Value=S*b
  S*cbar : Constant  Value=S*cbar
  W : Constant  Value=W
  Zeng : Constant  Value=Zeng
  b : Constant  Value=b
  b/2 : Constant  Value=b/2
  c : Constant  Value=c
  "cbar " : Constant  Value=cbar
  cmg : Constant  Value=194.9910
  cng : Constant  Value=187.1616
  kmg : Constant  Value=9499.1
  kng : Constant  Value=8716.2
  Vect_Costanti : Outport  VectorParamsAs1DForOutWhenUnconnected=off
  wires:
  "CY_p "/1 -> Bus Creator2/5  "CYp"
  Cl_dR/1 -> Bus Creator3/4  "CldR"
  "Cn_dR "/1 -> Bus Creator3/10  "CndR"
  "CL_q "/1 -> Bus Creator2/1  "CLq"
  "Cn_p "/1 -> Bus Creator3/8  "Cnp"
  Bus Creator1/1 -> Bus Creator5/2  "Coef_Propulsivi"
  CD_0/1 -> Bus Creator2/3  "CD0"
  Bus Creator4/1 -> Bus Creator5/3  "Coef_Aerodinamici"
  "Cm_dE "/1 -> Bus Creator3/6  "CmdE"
  "Cn_r "/1 -> Bus Creator3/7  "Cnr"
  "Cl_r "/1 -> Bus Creator3/2  "Clr"
  "Cm_q "/1 -> Bus Creator3/5  "Cmq"
  CY_dR/1 -> Bus Creator2/7  "CYdR"
  Cl_dA/1 -> Bus Creator3/3  "CldA"
  CY_dA/1 -> Bus Creator2/6  "CYdA"
  "CL_dE "/1 -> Bus Creator2/2  "CLdE"
  Dprop/1 -> Bus Creator/10  "Dprop"
  Cn_dA/1 -> Bus Creator3/9  "CndA"
  Bus Creator5/1 -> Vect_Costanti/1  "Costanti"
  Bus Creator/1 -> Bus Creator5/1  "Coef_Geometrici"
  Jeng/1 -> Bus Creator1/1  "Jeng"
  c/1 -> Bus Creator/1  "c"
  "S*b "/1 -> Bus Creator/6  "S*b"
  W/1 -> Bus Creator/8  "W"
  Rprop/1 -> Bus Creator/9  "Rprop"
  b/1 -> Bus Creator/3  "b"
  Bus Creator3/1 -> Bus Creator4/2  "Coef_Momenti"
  Bus Creator2/1 -> Bus Creator4/1  "Coef_Forze"
  S*cbar/1 -> Bus Creator/7  "S*cbar"
  Jprop/1 -> Bus Creator1/2  "Jprop"
  b/2/1 -> Bus Creator/4  "b/2"
  "Cl_p "/1 -> Bus Creator3/1  "Clp"
  CY_r/1 -> Bus Creator2/4  "CYr"
  S/1 -> Bus Creator/5  "S"
  "cbar "/1 -> Bus Creator/2  "cbar"
  Zeng/1 -> Bus Creator1/3  "Zeng"
  Constant/1 -> Bus Creator6/1  "rPG"
  Bus Creator6/1 -> Bus Creator5/4  "Vett_caratteristici"
  Constant3/1 -> Bus Creator6/4  "rmglG"
  Constant8/1 -> Bus Creator6/8  "rNPG"
  Constant6/1 -> Bus Creator6/7  "rACwG"
  Constant5/1 -> Bus Creator6/6  "rLEG"
  Constant4/1 -> Bus Creator6/5  "rngG"
  Constant7/1 -> Bus Creator6/9  "rACtG"
  Constant2/1 -> Bus Creator6/3  "rmgrG"
  Constant1/1 -> Bus Creator6/2  "rAHRSG"
  kng/1 -> Bus Creator7/1  "kng"
  kmg/1 -> Bus Creator7/2  "kmg"
  cng/1 -> Bus Creator7/3  "cng"
  cmg/1 -> Bus Creator7/4  "cmg"
  Bus Creator7/1 -> Bus Creator5/5  "gear"

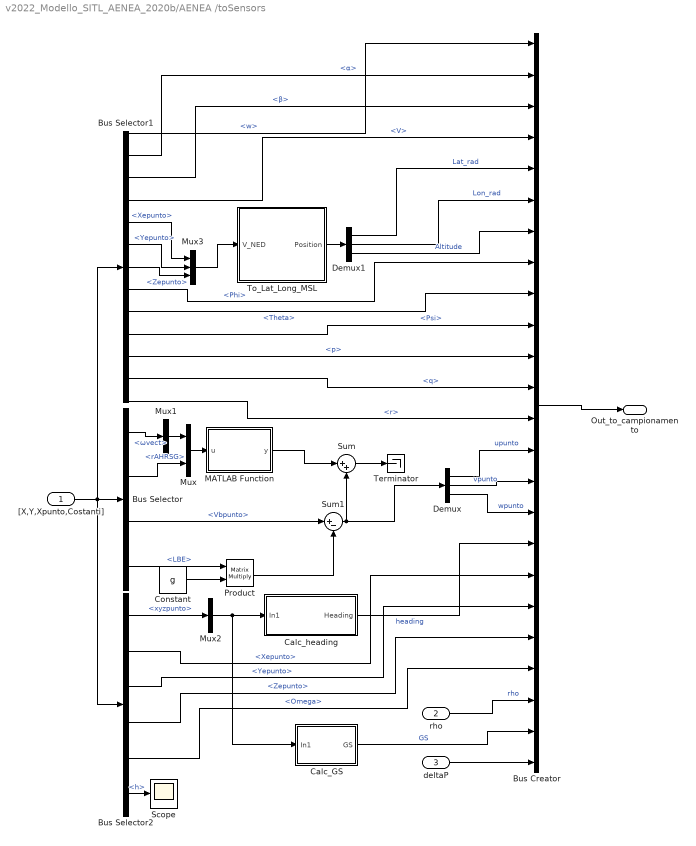
== system v2022_Modello_SITL_AENEA_2020b/AENEA /toSensors ==
  "[X,Y,Xpunto,Costanti]" : Inport
  rho : Inport  Port=2
  deltaP : Inport  Port=3
  Bus Creator : BusCreator  Inputs=24
  Bus Selector : BusSelector  OutputSignals=X.ωvect,Costanti.Vett_caratteristici.rAHRSG,Xpunto.Vbpunto,Y.LBE
  Bus Selector1 : BusSelector  OutputSignals=X.uvw.w,Y.Vbpolare.α,Y.Vbpolare.β,Y.Vbpolare.V,Xpunto.xyzpunto.Xepunto,Xpunto.xyzpunto.Yepunto,Xpunto.xyzpunto.Zepunto,X.PhiThetaPsi.Phi,X.PhiThetaPsi.Theta,X.PhiThetaPsi.Psi,X.ωvect.p,X.ωvect.q,X.ωvect.r
  Bus Selector2 : BusSelector  OutputSignals=Xpunto.xyzpunto,Xpunto.xyzpunto.Xepunto,Xpunto.xyzpunto.Yepunto,Xpunto.xyzpunto.Zepunto,Y.Omega,X.xyz.h
  Calc_GS : Subsystem
  Calc_heading : Subsystem
  Constant : Constant  Value=g
  Demux : Demux  Outputs=3
  Demux1 : Demux  Outputs=3
  MATLAB Function : MATLAB Function  TreatAsAtomicUnit=on
  Mux : Mux  Inputs=2
  Mux1 : Mux  Inputs=1
  Mux2 : Mux  Inputs=1
  Mux3 : Mux  Inputs=3
  Product : Product  Multiplication=Matrix(*)
  Scope : Scope
  Sum : Sum  Inputs=|++
  Sum1 : Sum  Inputs=|+-
  Terminator : Terminator
  To_Lat_Long_MSL : Subsystem
  Out_to_campionamento : Outport  VectorParamsAs1DForOutWhenUnconnected=off
  wires:
  "[X,Y,Xpunto,Costanti]"/1 -> Bus Selector2/1, Bus Selector1/1, Bus Selector/1
  Mux/1 -> MATLAB Function/1(u)
  Mux1/1 -> Mux/1
  Bus Selector/4 -> Product/1  "<LBE>"
  Constant/1 -> Product/2
  Mux2/1 -> Calc_GS/1(In1), Calc_heading/1(In1)
  Bus Selector2/1 -> Mux2/1  "<xyzpunto>"
  Bus Selector1/1 -> Bus Creator/1  "<w>"
  Bus Selector1/2 -> Bus Creator/2  "<α>"
  Bus Selector1/3 -> Bus Creator/3  "<β>"
  Bus Creator/1 -> Out_to_campionamento/1
  Bus Selector1/4 -> Bus Creator/4  "<V>"
  Bus Selector1/8 -> Bus Creator/8  "<Phi>"
  Bus Selector1/9 -> Bus Creator/9  "<Theta>"
  Bus Selector1/10 -> Bus Creator/10  "<Psi>"
  Bus Selector1/11 -> Bus Creator/11  "<p>"
  Bus Selector1/12 -> Bus Creator/12  "<q>"
  Bus Selector1/13 -> Bus Creator/13  "<r>"
  Demux/1 -> Bus Creator/14  "upunto"
  Demux/2 -> Bus Creator/15  "vpunto"
  Demux/3 -> Bus Creator/16  "wpunto"
  Calc_heading/1(Heading) -> Bus Creator/17  "heading"
  Bus Selector2/5 -> Bus Creator/21  "<Omega>"
  rho/1 -> Bus Creator/22  "rho"
  Calc_GS/1(GS) -> Bus Creator/23  "GS"
  Mux3/1 -> To_Lat_Long_MSL/1(V_NED)
  Bus Selector1/7 -> Mux3/3  "<Zepunto>"
  Bus Selector1/6 -> Mux3/2  "<Yepunto>"
  Bus Selector1/5 -> Mux3/1  "<Xepunto>"
  To_Lat_Long_MSL/1(Position) -> Demux1/1
  Demux1/1 -> Bus Creator/5  "Lat_rad"
  Demux1/2 -> Bus Creator/6  "Lon_rad"
  Demux1/3 -> Bus Creator/7  "Altitude"
  Bus Selector2/2 -> Bus Creator/18  "<Xepunto>"
  Bus Selector2/3 -> Bus Creator/19  "<Yepunto>"
  Bus Selector2/4 -> Bus Creator/20  "<Zepunto>"
  Bus Selector/1 -> Mux1/1  "<ωvect>"
  Bus Selector/2 -> Mux/2  "<rAHRSG>"
  MATLAB Function/1(y) -> Sum/1
  Sum/1 -> Terminator/1
  Product/1 -> Sum1/2
  Bus Selector2/6 -> Scope/1  "<h>"
  Sum1/1 -> Demux/1, Sum/2
  Bus Selector/3 -> Sum1/1  "<Vbpunto>"
  deltaP/1 -> Bus Creator/24

== system v2022_Modello_SITL_AENEA_2020b/Ricezione segnali2/Subsystem1 ==
  In1 : Inport
  In2 : Inport  Port=2
  In3 : Inport  Port=3
  In4 : Inport  Port=4
  AILERON : Subsystem
  Degrees to Radians : simulink_extras/Transformations/Degrees to Radians
  Degrees to Radians1 : simulink_extras/Transformations/Degrees to Radians
  Degrees to Radians2 : simulink_extras/Transformations/Degrees to Radians
  ELEVATOR : Subsystem
  RUDDER : Subsystem
  Scope : Scope  NumInputPorts=2
  Scope1 : Scope
  Scope2 : Scope  NumInputPorts=2
  Scope3 : Scope
  Scope4 : Scope
  THROTTLE : Subsystem
  Out1 : Outport  VectorParamsAs1DForOutWhenUnconnected=off
  Out2 : Outport  Port=2  VectorParamsAs1DForOutWhenUnconnected=off
  Out3 : Outport  Port=3  VectorParamsAs1DForOutWhenUnconnected=off
  Out4 : Outport  Port=4  VectorParamsAs1DForOutWhenUnconnected=off
  wires:
  In3/1 -> AILERON/1(In1)
  In4/1 -> RUDDER/1(In1)
  In2/1 -> Scope/1, ELEVATOR/1(In1)
  In1/1 -> Scope2/1, THROTTLE/1(In1)
  Degrees to Radians2/1 -> Out4/1, Scope4/1  "Timone"
  Degrees to Radians1/1 -> Out3/1, Scope3/1  "Alettoni"
  Degrees to Radians/1 -> Scope/2, Scope1/1, Out2/1  "Equilibratore"
  THROTTLE/1(Out1) -> Scope2/2, Out1/1  "Manetta"
  ELEVATOR/1(Out1) -> Degrees to Radians/1  "Equilibratore"
  AILERON/1(Out1) -> Degrees to Radians1/1  "Alettoni"
  RUDDER/1(Out1) -> Degrees to Radians2/1  "Timone"
